simulink model "Simulink1"  (R2019b)
settings: Solver=FixedStepAuto  StartTime=0.0  StopTime=10.0  RelTol=1e-3  EnableMultiTasking=on
libraries: legoev3lib x2
settings Model: ExtModeTrigDuration=2  Creator=nikit  LastModifiedBy=nikit
settings SolverCC: PositivePriorityOrder=on
settings OptimizationCC: EnhancedBackFolding=on  PassReuseOutputArgsAs=Individual arguments  ZeroExternalMemoryAtStartup=off  ZeroInternalMemoryAtStartup=off  MaxStackSize=64  OptimizeBlockOrder=speed  DifferentSizesBufferReuse=on  OptimizationCustomize=off  EfficientTunableParamExpr=on
settings DebuggingCC: ParameterTunabilityLossMsg=error
settings HardwareCC: ProdBitPerPointer=32  ProdBitPerSizeT=32  ProdBitPerPtrDiffT=32  ProdLargestAtomicInteger=Long  ProdWordSize=32  ProdHWDeviceType=ARM Compatible->ARM 9
settings SFSimCC: MATLABDynamicMemAlloc=off
settings RTWCC: SystemTargetFile=ert.tlc  HardwareBoard=LEGO MINDSTORMS EV3  TLCOptions="-aInlineSetEventsForThisBaseRateFcn=TLC_FALSE -aSuppressMultiTaskScheduler=TLC_FALSE  -aRateBasedStepFcn=0"  TemplateMakefile=ert_default_tmf  GenerateReport=on  Toolchain=Sourcery G++ Lite v2009q3  IncludeHyperlinkInReport=on  LaunchReport=on  GenerateTraceInfo=on  GenerateTraceReport=on  GenerateTraceReportSl=on  GenerateTraceReportSf=on  GenerateTraceReportEml=on
settings CodeAppCC: ForceParamTrailComments=on  IgnoreCustomStorageClasses=off  OperatorAnnotations=on  SimulinkDataObjDesc=on  SFDataObjDesc=on  InsertBlockDesc=on
settings ERTTargetCC: SupportContinuousTime=on  SupportVariableSizeSignals=on

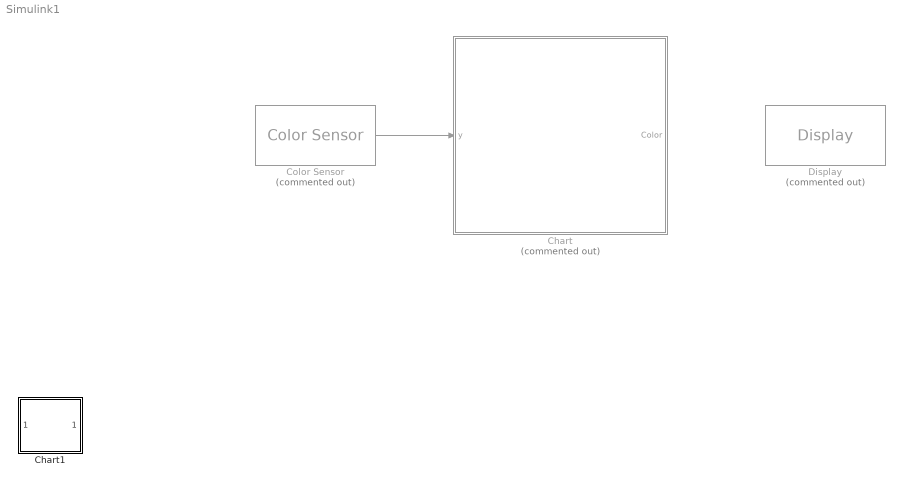
== system Simulink1 ==
  Chart : Stateflow chart  Commented=on  BlockKeywords=__PRM__SERIALIZED__DATA__:Stateflow Chart,Stateflow Diagram  TreatAsAtomicUnit=on
  Chart1 : Stateflow chart  BlockKeywords=__PRM__SERIALIZED__DATA__:Stateflow Chart,Stateflow Diagram  TreatAsAtomicUnit=on
  Color Sensor : legoev3lib/Color Sensor  Commented=on  portNumber=2  mode=Color  sampleTime=0.5
      settings: SourceProductName=Simulink Support Package for LEGO MINDSTORMS EV3 Hardware  SourceProductBaseCode=LEGOEV3
  Display : legoev3lib/Display  Commented=on  slcdStr=Color  slcdLine=1  slcdFormat=Hex
      settings: SourceProductName=Simulink Support Package for LEGO MINDSTORMS EV3 Hardware  SourceProductBaseCode=LEGOEV3
  wires:
  Color Sensor/1 -> Chart/1(y)
  ? -> Display/1

== stateflow chart Simulink1/Chart1 ==
  state Default
    color_code=0;
  state Check_1
    color_code=1;
  state Check_6
    color_code=6;
  (default) -> Default
  Default -> Check_1 [order 1] : [sns_val ==1]
  Default -> Check_6 [order 2] : [sns_val ==6]
  Check_1 -> Default [order 2] : [(sns_val ~= 1) & (sns_val ~=6) ]
  Check_6 -> Default [order 2] : [(sns_val ~= 1) & (sns_val ~=6)]
  Check_6 -> Check_1 [order 1] : [sns_val ==1]
  Check_1 -> Check_6 [order 1] : [sns_val==6]
  data: sns_val input; color_code output

== stateflow chart Simulink1/Chart ==
  state BLACK
    Color = "Black";
  state WHITE
    Color = "White";
  (default) -> BLACK
  BLACK -> WHITE : [y ==6]
  WHITE -> BLACK : [y == 1]
  data: y input; Color output Enum: ChartModeType
